simulink model "Convolution_Stream_Ex1"  (R2024a)
settings: Solver=VariableStepAuto  StartTime=0.0  StopTime=256  RelTol=1e-3
InitFcn:
  | F_Length = 32;
  | G_Length = 16;
undefined symbols (not defined in the file): S, vsva2197, xcvc1902
libraries: aieDSP x1, vmcUtilities x1
settings Model: Creator=sdegala  LastModifiedBy=sdegala
settings ModelReferenceCC: EnableRefExpFcnMdlSchedulingChecks=on
settings RTWCC: GPUComputeCapability=3.5
settings ConfigComp: CovBoundaryAbsTol=1.0e-5

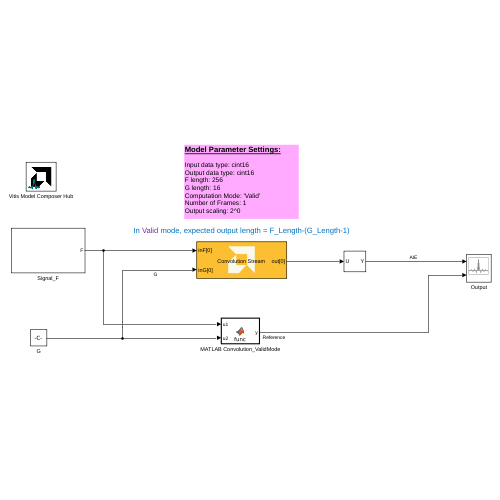
[thumbnail: Simulink's stored preview of the top-level diagram]
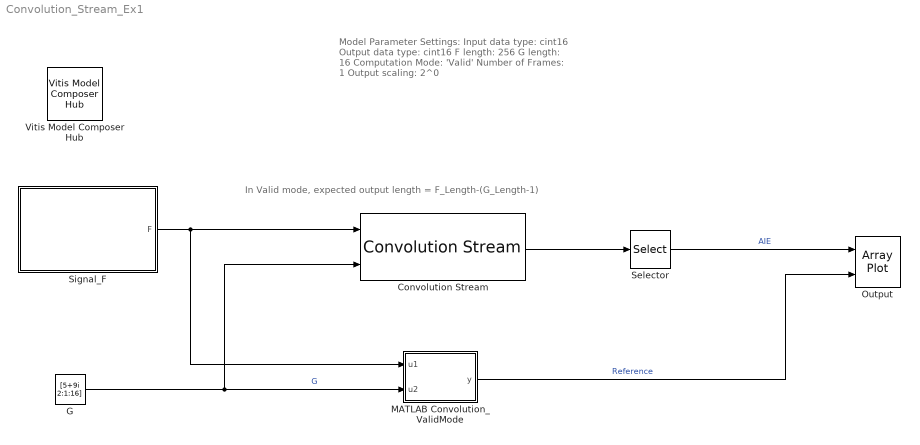
== system Convolution_Stream_Ex1 ==
  note: In Valid mode, expected output length = F_Length-(G_Length-1)
  note: Model Parameter Settings:
      |
      | Input data type: cint16
      | Output data type: cint16
      | F length: 256
      | G length: 16
      | Computation Mode: 'Valid'
      | Number of Frames: 1
      | Output scaling: 2^0
  Convolution Stream : aieDSP/Convolution Stream  AIE_VARIANT=1  api=1  data_type_f=cint16  data_type_g=cint16  data_type_out=cint16  function_type=1  compute_mode=Valid  f_sample_size=256  g_sample_size=16  USE_RTP_VECTOR_LENGTHS=off  num_frames=1  shift_output=0  rnd_mode=Floor  sat_mode=None  no_of_kernels=1  casc_length=1  blockJsonConstraints=[]  blockJsonConstraintsInternal=[]  spec=vmc_stream_conv.json  SerializedMaskParamNames=[]  SerializedMaskParamValues=[]  SerializedMaskParamVisibilities=[]  block_type=Convolution Stream  SerializedMaskParamDataypes=uint|uint|typename|typename|typename|uint|uint|uint|uint|uint|uint|uint|uint|uint|uint|uint  SerializedMaskParamEnumStrArr=0|0|0|0|0|0|Full,Same,Valid|0|0|0|0|0|Floor,Ceiling,Round to positive infinity,Round to negative infinity,Round symmetrical to infinity,Round symmetrical to zero,Round convergent to even,Round convergent to odd|None,Saturate,Symmetric|0|0  SerializedMaskParamEnumValArr=0|0|0|0|0|0|0,1,2|0|0|0|0|0|0,1,2,3,4,5,6,7|0,1,3|0|0  SerializedMaskParamVectorArr=0|0|0|0|0|0|0|0|0|0|0|0|0|0|0|0  SerializedMaskParamKeys=AIE_VARIANT|TP_API|TT_DATA_F|TT_DATA_G|TT_DATA_OUT|TP_FUNCT_TYPE|TP_COMPUTE_MODE|TP_F_LEN|TP_G_LEN|TP_USE_RTP_VECTOR_LENGTHS|TP_NUM_FRAMES|TP_SHIFT|TP_RND|TP_SAT|TP_PHASES|TP_CASC_LEN
  G : Constant  Value=[5+9i 2:1:16]  OutDataTypeStr=int16  SampleTime=1
  MATLAB Convolution_ValidMode : MATLAB Function  TreatAsAtomicUnit=on
  Output : ArrayPlot  NumInputPorts=2  WindowPosition=[560.000000,350.000000,800.000000,500.000000,]  Visible=on  ScopeFrameLocation=window  YLimits=[-3923.75 36843.75]  ShowLegend=on
  Selector : Selector  InputPortWidth=241  IndexOptions=Index vector (dialog)  Indices=17:1:241  OutputSizes=1
  Signal_F : Subsystem
  Vitis Model Composer Hub : vmcUtilities/Vitis Model Composer Hub  Tag=genX  CodeGeneration=off  StartColumn=1  NumberOfColumns=1  TargetDirectory=./code  exportDesign=off  analyzeDesign=off  validateDesignOnHw=off  ExportType=AI Engines  IpVendor=xilinx.com  IpLibrary=hls  IpVersion=1.0  IpHWLanguage=Verilog  AieCompilerOptions={}  AieSimulatorOptions={}  CreateTestbench=off  TestbenchStackSize=10  RunRtlSim=off  RunCSim=off  RunAieSim=off  AieSimTimeout=50000  RunAieSimProfiling=off  LaunchVitisAnalyzer=off  PlotOutput=off  RunX86Sim=off  X86SimTimeout=10  GenHwImage=off  GenLibadfXo=off  GenHwValidationCode=off  PlatformType=Not Specified  HwSystemType=Baremetal  HwValidationTarget=hw  ProjDevice=xcvc1902-vsva2197-1LP-e-S  ProjDevicePart=xcvc1902-vsva2197-1LP-e-S  AIEType=AIE  SamplePeriod=-1  ClockFrequency=200  DataPathParallelism=1  xilinxfamily=versalaicore  part=xcvc1902  speed=-1LP-e-S  package=vsva2197  directory=./netlist  testbench=off  incr_netlist=off  synthesis_tool=Vivado  clock_wrapper=Clock Enables  dbl_ovrd=According to Block Masks  dcm_input_clock_period=10  sysclk_period=10  simulink_period=1  eval_field=0  LogFileName=''  NThreads=4
  wires:
  MATLAB Convolution_ValidMode/1(y) -> Output/2  "Reference"
  Convolution Stream/1 -> Selector/1
  G/1 -> Convolution Stream/2, MATLAB Convolution_ValidMode/2(u2)  "G"
  Signal_F/1(F) -> Convolution Stream/1, MATLAB Convolution_ValidMode/1(u1)
  Selector/1 -> Output/1  "AIE"

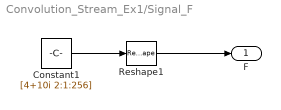
== system Convolution_Stream_Ex1/Signal_F ==
  Constant1 : Constant  Value=[4+10i 2:1:256]  OutDataTypeStr=int16  SampleTime=1
  Reshape1 : Reshape
  F : Outport
  wires:
  Constant1/1 -> Reshape1/1
  Reshape1/1 -> F/1

== matlab function Convolution_Stream_Ex1/MATLAB Convolution_ValidMode ==
  data: u1 input; y output; u2 input
function y = func(u1,u2)

y = int16(conv(u1,u2,"valid"));
